simulink model "Guidance_PC_07Mar2013"  (Simulink 7.7)
settings: Solver=ode4  StartTime=0.0  StopTime=inf  FixedStep=sample_time  RelTol=1e-3
InitFcn:
  | sample_time=0.02;
undefined symbols (not defined in the file or in its folder): DiscIntNeverNeededParam
libraries: simulink x6, utility x1
(part 1 of 2)
settings Model: Creator=ttcl3  LastModifiedBy=Zhao Weihua
settings SolverCC: MaxConsecutiveMinStep=auto
settings DebuggingCC: MultiTaskRateTransMsg=warning

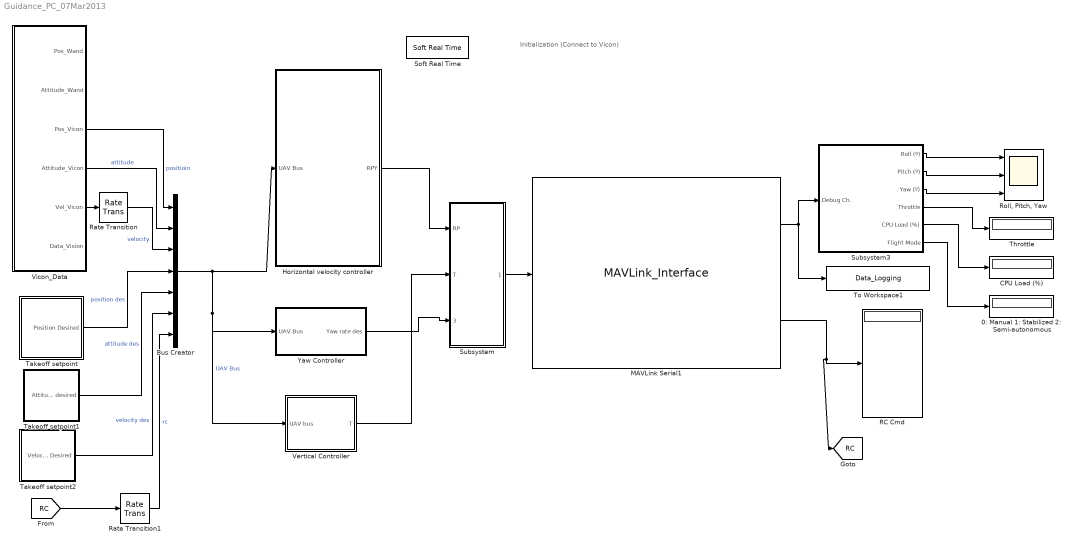
== system Guidance_PC_07Mar2013 ==
  note: Initialization
      | (Connect to Vicon)
  0: Manual 1: Stabilized 2: Semi-autonomous : Display
  Bus Creator : BusCreator  Inputs=7
  CPU Load (%) : Display
  Horizontal velocity controller : Subsystem
  MAVLink Serial1 : S-Function  FunctionName=MAVLink_Interface  Parameters=COM_Port,Baud_Rate,MSG_INPUT,MSG_OUTPUT  EnableBusSupport=off  mask{COM_Port='COM8', Baud_Rate=57600, HEART_BEAT=off, ATTITUDE_OUT=on, RAW_IMU=off, POSITION_OUT=off, VFR_HUD=off, RC_SCALED=on, SERVO_OUT_RAW=off, VICON_XYZ_RPY_Output=off, SET_MODE=off, DATA_STREAM=off, ATTITUDE_COMMAND=off, ATTITUDE_IN=off, GPS_RAW_IN=off, VFR_HUD_IN=off, VICON_XYZ_RPY=on, VICON_VEL=off, POSITION_DESIRED=off}
      mask prompts: COM_Port "COM Port"; Baud_Rate "Baud Rate"; HEART_BEAT "HEART BEAT"; ATTITUDE_OUT "ATTITUDE"; RAW_IMU "RAW IMU"; POSITION_OUT "GLOBAL POSITION"; VFR_HUD "VFR HUD"; RC_SCALED "RC CHANNELS SCALED"; SERVO_OUT_RAW "SERVO OUTPUT RAW"; VICON_XYZ_RPY_Output "VICON Output"; SET_MODE "SET MODE"; DATA_STREAM "REQUEST DATA STREAM"; ATTITUDE_COMMAND "ATTITUDE COMMAND"; ATTITUDE_IN "ATTITUDE (HIL)"; GPS_RAW_IN "GPS RAW (HIL)"; VFR_HUD_IN "AIRSPEED (HIL)"; VICON_XYZ_RPY "VICON POSITION"; VICON_VEL "VICON SPEED"; POSITION_DESIRED "Position Desired"
      mask init:
      | MSG_ID_NUM_INPUT = [uint8(11) uint8(66) uint8(59) uint8(30) uint8(32) uint8(73) uint8(104) uint8(103) uint8(50)];
      | MSG_ID_NAME_INPUT = [SET_MODE DATA_STREAM ATTITUDE_COMMAND ATTITUDE_IN GPS_RAW_IN VFR_HUD_IN VICON_XYZ_RPY VICON_VEL POSITION_DESIRED];
      | 
      | MSG_ID_NUM_OUTPUT = [uint8(0) uint8(30) uint8(27) uint8(73) uint8(74) uint8(34) uint8(37) uint8(104)];
      | MSG_ID_NAME_OUTPUT = [HEART_BEAT ATTITUDE_OUT RAW_IMU VFR_HUD POSITION_OUT RC_SCALED SERVO_OUT_RAW VICON_XYZ_RPY_Output];
      | 
      | idx_input = find(MSG_ID_NAME_INPUT);
      | MSG_INPUT = MSG_ID_NUM_INPUT(idx_input);
      | 
      | idx_output = find(MSG_ID_NAME_OUTPUT);
      | MSG_OUTPUT = MSG_ID_NUM_OUTPUT(idx_output);
      mask TabNameString: Setting,Setting,Output Message,Output Message,Output Message,Output Message,Output Message,Output Message,Output Message,Output Message,Input Message,Input Message,Input Message,Input Message,Input Message,Input Message,Input Message,Input Message,Input Message
      mask Display:
      | % Block image
      | image(imread('10-inch Quad Heat Map.png'));
      | 
      | %Label block
      | fprintf('MAVLink Serial\n%s\n%dbps', COM_Port,  Baud_Rate)
      | 
      | 
      | %Label input ports
      | 
      | in = 1;
      | if (SET_MODE == 1)
      |     port_label('input', in, 'SET MODE');
      |     in = in + 1;
      | end
      | if (DATA_STREAM == 1)
      |     port_label('input', in, 'REQUEST DATA STREAM');
      |     in = in + 1;
      | end
      | if (ATTITUDE_COMMAND == 1)
      |     port_label('input', in, 'ATTITUDE COMMAND');
      |     in = in + 1;
      | end
      | if (ATTITUDE_IN == 1)
      |     port_label('input', in, 'ATTITUDE (HIL)');
      |     in = in + 1;
      | end
      | if (GPS_RAW_IN == 1)
      |     port_label('input', in, 'GPS RAW (HIL)');
      |     in = in + 1;
      | end
      | if (VFR_HUD_IN == 1)
      |     port_label('input', in, 'AIRSPEED (HIL)');
      |     in = in + 1;
      | end
      | if (VICON_XYZ_RPY == 1)
      |     port_label('input', in, 'RPYT CMD');
      |     in = in + 1;
      | end
      | if (VICON_VEL == 1)
      |     port_label('input', in, 'VICON_VEL');
      |     in = in + 1;
      | end
      | 
      | if (POSITION_DESIRED == 1)
      |     port_label('input', in, 'POSITION_DESIRED');
      |     in = in + 1;
      | end
      | 
      | %Label output ports
      | 
      | out = 1;
      | if (HEART_BEAT == 1)
      |     port_label('output', out, 'HEART BEAT');
      |     out = out + 1;
      | end
      | if (ATTITUDE_OUT == 1)
      |     port_label('output', out, 'DEBUG');
      |     out = out + 1;
      | end
      | if (RAW_IMU == 1)
      |     port_label('output', out, 'RAW IMU');
      |     out = out + 1;
      | end
      | if (POSITION_OUT == 1)
      |     port_label('output', out, 'GLOBAL POSITION');
      |     out = out + 1;
      | end
      | if (VFR_HUD == 1)
      |     port_label('output', out, 'VFR HUD');
      |     out = out + 1;
      | end
      | if (RC_SCALED == 1)
      |     port_label('output', out, 'RC CMD');
      |     out = out + 1;
      | end
      | if (SERVO_OUT_RAW == 1)
      |     port_label('output', out, 'SERVO OUTPUT RAW');
      |     out = out + 1;
      | end
      | % weihua, vicon output
      | if (VICON_XYZ_RPY_Output == 1)
      |     port_label('output', out, 'VICON_XYZ_RPY');
      |     out = out + 1;
      | end
  RC Cmd : Display
  Rate Transition : RateTransition  OutPortSampleTime=sample_time
  Rate Transition1 : RateTransition  OutPortSampleTime=sample_time
  "Roll, Pitch, Yaw" : Scope  NumInputPorts=3
      settings: TickLabels=on  TimeRange=60  YMin=-1~-0.1~-1  YMax=1~0.1~1  SampleInput=on
  Soft Real Time : utility/Soft Real Time  x=0.6
  Subsystem : Subsystem
  Subsystem3 : Subsystem
  Takeoff setpoint : Subsystem
  Takeoff setpoint1 : Subsystem
  Takeoff setpoint2 : Subsystem
  Throttle : Display
  To Workspace1 : ToWorkspace  VariableName=Data_Logging  SampleTime=-1  SaveFormat=Structure With Time
  Vertical Controller : Subsystem
  Vicon_Data : Subsystem
  Yaw Controller : Subsystem
  tag scope: RC=global
  wires:
  MAVLink Serial1/2 -> RC Cmd/1, [RC]
  Subsystem3/1(Roll (º)) -> "Roll, Pitch, Yaw"/1
  Subsystem3/2(Pitch (º)) -> "Roll, Pitch, Yaw"/2
  Subsystem3/3(Yaw (º)) -> "Roll, Pitch, Yaw"/3
  Subsystem3/4(Throttle) -> Throttle/1
  Subsystem3/5(CPU Load (%)) -> CPU Load (%)/1
  Subsystem3/6(Flight Mode) -> 0: Manual 1: Stabilized 2: Semi-autonomous/1
  MAVLink Serial1/1 -> Subsystem3/1(Debug Ch.), To Workspace1/1
  Vicon_Data/5(Vel_Vicon) -> Rate Transition/1
  [RC] -> Rate Transition1/1
  Horizontal velocity controller/1(RPY) -> Subsystem/1(RP)
  Subsystem/1(XYZ RPY) -> MAVLink Serial1/1
  Vicon_Data/3(Pos_Vicon) -> Bus Creator/1  "positioin"
  Vicon_Data/4(Attitude_Vicon) -> Bus Creator/2  "attitude"
  Rate Transition/1 -> Bus Creator/3  "velocity"
  Takeoff setpoint/1(Position Desired) -> Bus Creator/4  "position des"
  Takeoff setpoint1/1(Attitude desired) -> Bus Creator/5  "attitude des"
  Takeoff setpoint2/1(Velocity Desired) -> Bus Creator/6  "velocity des"
  Rate Transition1/1 -> Bus Creator/7  "rc"
  Bus Creator/1 -> Horizontal velocity controller/1(UAV Bus), Yaw Controller/1(UAV Bus), Vertical Controller/1(UAV bus)  "UAV Bus"
  Yaw Controller/1(Yaw rate des) -> Subsystem/3(Yaw rate)
  Vertical Controller/1(T) -> Subsystem/2(T)

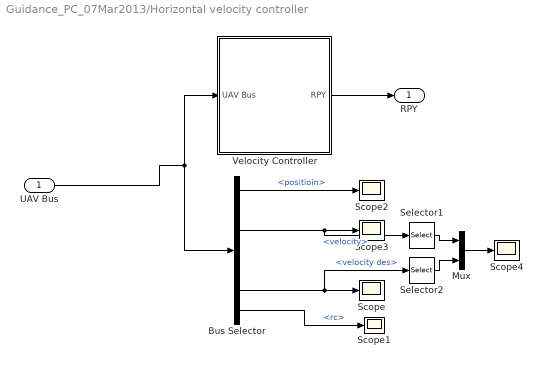
== system Guidance_PC_07Mar2013/Horizontal velocity controller ==
  UAV Bus : Inport
  Bus Selector : BusSelector  OutputSignals=positioin,attitude,velocity,position des,attitude des,velocity des,rc
  Mux : Mux  Inputs=2
  Scope{,1..4} (5 alike) : Scope
      Scope1 settings: SaveName=ScopeData2
      Scope2 settings: SaveName=ScopeData3
      Scope3 settings: SaveName=ScopeData6
      Scope4 settings: SaveName=ScopeData7
  Selector1 : Selector  InputPortWidth=3  IndexOptions=Index vector (dialog)  Indices=[2]  OutputSizes=1
  Selector2 : Selector  InputPortWidth=3  IndexOptions=Index vector (dialog)  Indices=[2]  OutputSizes=1
  Velocity Controller : Subsystem
  RPY : Outport
  wires:
  UAV Bus/1 -> Velocity Controller/1(UAV Bus), Bus Selector/1
  Velocity Controller/1(RPY) -> RPY/1
  Bus Selector/6 -> Scope/1, Selector2/1  "<velocity des>"
  Bus Selector/7 -> Scope1/1  "<rc>"
  Bus Selector/1 -> Scope2/1  "<positioin>"
  Bus Selector/3 -> Scope3/1, Selector1/1  "<velocity>"
  Selector1/1 -> Mux/1
  Selector2/1 -> Mux/2
  Mux/1 -> Scope4/1

== system Guidance_PC_07Mar2013/Subsystem ==
  note: 7x1 vector (usec, XYZRPY)
  RP : Inport
  T : Inport  Port=2
  Yaw rate : Inport  Port=3
  Mux1 : Mux  Inputs=3
  Mux2 : Mux  Inputs=3
  Mux3 : Mux  Inputs=2
  usec : Constant  Value=0
  XYZ RPY : Outport
  wires:
  Mux1/1 -> XYZ RPY/1
  usec/1 -> Mux1/1, Mux2/1, Mux2/2
  Mux2/1 -> Mux1/2
  T/1 -> Mux2/3
  RP/1 -> Mux3/1
  Yaw rate/1 -> Mux3/2
  Mux3/1 -> Mux1/3

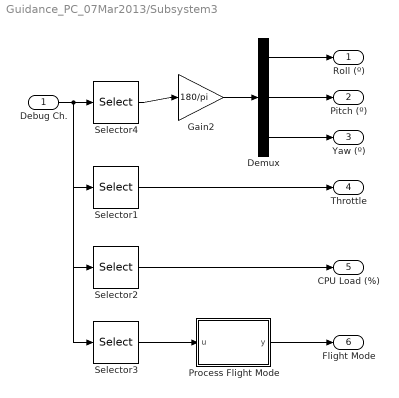
== system Guidance_PC_07Mar2013/Subsystem3 ==
  Debug Ch. : Inport
  Demux : Demux  Outputs=3
  Gain2 : Gain  Gain=180/pi
  Process Flight Mode : Stateflow chart  TreatAsAtomicUnit=on
  Selector1 : Selector  InputPortWidth=6  IndexOptions=Index vector (dialog)  Indices=4  OutputSizes=1
  Selector2 : Selector  InputPortWidth=6  IndexOptions=Index vector (dialog)  Indices=5  OutputSizes=1
  Selector3 : Selector  InputPortWidth=6  IndexOptions=Index vector (dialog)  Indices=6  OutputSizes=1
  Selector4 : Selector  InputPortWidth=6  IndexOptions=Index vector (dialog)  Indices=[1 2 3]  OutputSizes=1
  Roll (º) : Outport
  Pitch (º) : Outport  Port=2
  Yaw (º) : Outport  Port=3
  Throttle : Outport  Port=4
  CPU Load (%) : Outport  Port=5
  Flight Mode : Outport  Port=6
  wires:
  Selector4/1 -> Gain2/1
  Gain2/1 -> Demux/1
  Demux/1 -> Roll (º)/1
  Demux/2 -> Pitch (º)/1
  Debug Ch./1 -> Selector4/1, Selector1/1, Selector2/1, Selector3/1
  Demux/3 -> Yaw (º)/1
  Selector1/1 -> Throttle/1
  Selector2/1 -> CPU Load (%)/1
  Selector3/1 -> Process Flight Mode/1(u)
  Process Flight Mode/1(y) -> Flight Mode/1

== system Guidance_PC_07Mar2013/Takeoff setpoint ==
  Des_X : Constant  Value=0  SampleTime=sample_time
  Des_Y : Constant  Value=0  SampleTime=sample_time
  Des_Z : Constant  Value=-0.8  SampleTime=sample_time
  Mux3 : Mux  Inputs=3
  Position Desired : Outport
  wires:
  Des_X/1 -> Mux3/1
  Des_Y/1 -> Mux3/2
  Des_Z/1 -> Mux3/3
  Mux3/1 -> Position Desired/1

== system Guidance_PC_07Mar2013/Takeoff setpoint1 ==
  Mux3 : Mux  Inputs=3
  Pitch : Constant  Value=0  SampleTime=sample_time
  Roll : Constant  Value=0  SampleTime=sample_time
  Yaw : Constant  Value=0  OutDataTypeStr=double  SampleTime=sample_time
  Attitude desired : Outport
  wires:
  Mux3/1 -> Attitude desired/1
  Yaw/1 -> Mux3/3
  Pitch/1 -> Mux3/2
  Roll/1 -> Mux3/1

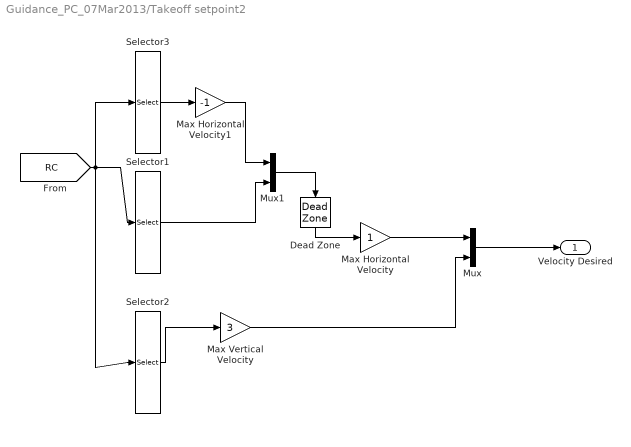
== system Guidance_PC_07Mar2013/Takeoff setpoint2 ==
  Dead Zone : DeadZone  LowerValue=-0.1  UpperValue=0.1  SaturateOnIntegerOverflow=on
  Max Horizontal Velocity : Gain  SampleTime=sample_time
  Max Horizontal Velocity1 : Gain  Gain=-1  OutDataTypeStr=double  SampleTime=sample_time
  Max Vertical Velocity : Gain  Gain=3  SampleTime=sample_time
  Mux : Mux  Inputs=2
  Mux1 : Mux  Inputs=2
  Selector1 : Selector  InputPortWidth=8  IndexOptions=Index vector (dialog)  Indices=[2]  OutputSizes=1
  Selector2 : Selector  InputPortWidth=8  IndexOptions=Index vector (dialog)  Indices=[1]  OutputSizes=1
  Selector3 : Selector  InputPortWidth=8  IndexOptions=Index vector (dialog)  Indices=[3]  OutputSizes=1
  Velocity Desired : Outport
  wires:
  [RC] -> Selector2/1, Selector1/1, Selector3/1
  Selector2/1 -> Max Vertical Velocity/1
  Mux/1 -> Velocity Desired/1
  Selector3/1 -> Max Horizontal Velocity1/1
  Selector1/1 -> Mux1/2
  Max Horizontal Velocity1/1 -> Mux1/1
  Mux1/1 -> Dead Zone/1
  Max Horizontal Velocity/1 -> Mux/1
  Max Vertical Velocity/1 -> Mux/2
  Dead Zone/1 -> Max Horizontal Velocity/1

== system Guidance_PC_07Mar2013/Vertical Controller ==
  UAV bus : Inport
  Bus Selector : BusSelector  OutputSignals=rc
  Selector2 : Selector  InputPortWidth=8  IndexOptions=Index vector (dialog)  Indices=[1]  OutputSizes=1
  T : Outport
  wires:
  UAV bus/1 -> Bus Selector/1
  Bus Selector/1 -> Selector2/1  "<rc>"
  Selector2/1 -> T/1

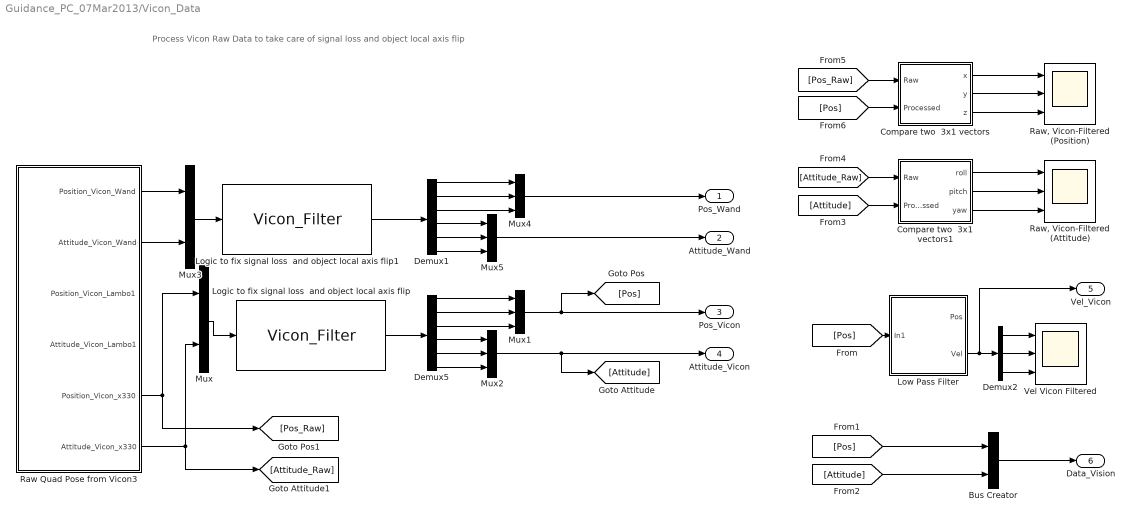
== system Guidance_PC_07Mar2013/Vicon_Data ==
  note: Process Vicon Raw Data to take care of signal loss and object local axis flip
  Bus Creator : BusCreator  Inputs=2
  Compare two  3x1 vectors : Subsystem
  Compare two  3x1 vectors1 : Subsystem
  Demux1 : Demux  Outputs=6
  Demux2 : Demux  Outputs=3
  Demux5 : Demux  Outputs=6
  Logic to fix signal loss  and object local axis flip : M-S-Function  FunctionName=Vicon_Filter
  Logic to fix signal loss  and object local axis flip1 : M-S-Function  FunctionName=Vicon_Filter
  Low Pass Filter : Subsystem
  Mux : Mux  Inputs=2
  Mux{1..2,4..5} (4 alike) : Mux  Inputs=3
  Mux3 : Mux  Inputs=2
  Raw Quad Pose from Vicon3 : Subsystem
  "Raw, Vicon-Filtered (Attitude)" : Scope  NumInputPorts=3
      settings: TimeRange=50  YMin=-3.14159~-1~-3.5  YMax=3.14159~1~3.5  SaveName=ScopeData4
  "Raw, Vicon-Filtered (Position)" : Scope  NumInputPorts=3
      settings: TimeRange=50  YMin=-2.09~2.281~-0.0655  YMax=-2.055~2.293~-0.063  SaveName=ScopeData10
  "Vel Vicon Filtered " : Scope  NumInputPorts=3
      settings: YMin=-0.7~-1~-9  YMax=0.4~7.5~0.5  SaveName=ScopeData5
  Pos_Wand : Outport
  Attitude_Wand : Outport  Port=2
  Pos_Vicon : Outport  Port=3
  Attitude_Vicon : Outport  Port=4
  Vel_Vicon : Outport  Port=5
  Data_Vision : Outport  Port=6
  wires:
  Demux2/1 -> "Vel Vicon Filtered "/1
  Demux2/2 -> "Vel Vicon Filtered "/2
  Demux2/3 -> "Vel Vicon Filtered "/3
  Compare two  3x1 vectors/1(x) -> "Raw, Vicon-Filtered (Position)"/1
  Compare two  3x1 vectors/2(y) -> "Raw, Vicon-Filtered (Position)"/2
  Low Pass Filter/2(Vel) -> Demux2/1, Vel_Vicon/1
  Mux/1 -> Logic to fix signal loss  and object local axis flip/1
  Logic to fix signal loss  and object local axis flip/1 -> Demux5/1
  Demux5/1 -> Mux1/1
  Demux5/2 -> Mux1/2
  Demux5/3 -> Mux1/3
  Demux5/4 -> Mux2/1
  Demux5/5 -> Mux2/2
  Demux5/6 -> Mux2/3
  Mux2/1 -> Attitude_Vicon/1, [Attitude]
  [Pos] -> Low Pass Filter/1(In1)
  Compare two  3x1 vectors/3(z) -> "Raw, Vicon-Filtered (Position)"/3
  Compare two  3x1 vectors1/1(roll) -> "Raw, Vicon-Filtered (Attitude)"/1
  Compare two  3x1 vectors1/2(pitch) -> "Raw, Vicon-Filtered (Attitude)"/2
  Mux1/1 -> Pos_Vicon/1, [Pos]
  Compare two  3x1 vectors1/3(yaw) -> "Raw, Vicon-Filtered (Attitude)"/3
  [Attitude_Raw] -> Compare two  3x1 vectors1/1(Raw)
  [Attitude] -> Compare two  3x1 vectors1/2(Processed)
  [Pos_Raw] -> Compare two  3x1 vectors/1(Raw)
  [Pos] -> Compare two  3x1 vectors/2(Processed)
  [Pos] -> Bus Creator/1
  [Attitude] -> Bus Creator/2
  Bus Creator/1 -> Data_Vision/1
  Mux3/1 -> Logic to fix signal loss  and object local axis flip1/1
  Logic to fix signal loss  and object local axis flip1/1 -> Demux1/1
  Demux1/1 -> Mux4/1
  Demux1/2 -> Mux4/2
  Demux1/3 -> Mux4/3
  Demux1/4 -> Mux5/1
  Demux1/5 -> Mux5/2
  Demux1/6 -> Mux5/3
  Mux5/1 -> Attitude_Wand/1
  Mux4/1 -> Pos_Wand/1
  Raw Quad Pose from Vicon3/1(Position_Vicon_Wand) -> Mux3/1
  Raw Quad Pose from Vicon3/2(Attitude_Vicon_Wand) -> Mux3/2
  Raw Quad Pose from Vicon3/5(Position_Vicon_x330) -> Mux/1, [Pos_Raw]
  Raw Quad Pose from Vicon3/6(Attitude_Vicon_x330) -> Mux/2, [Attitude_Raw]

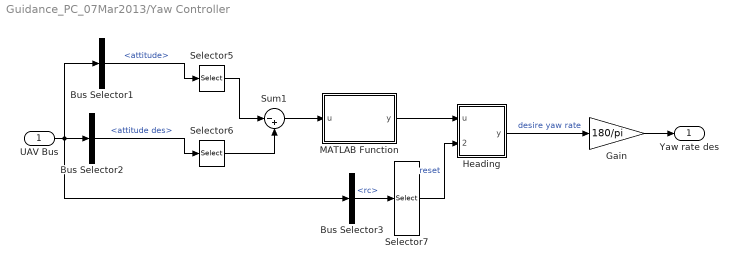
== system Guidance_PC_07Mar2013/Yaw Controller ==
  UAV Bus : Inport
  Bus Selector1 : BusSelector  OutputSignals=attitude
  Bus Selector2 : BusSelector  OutputSignals=attitude des
  Bus Selector3 : BusSelector  OutputSignals=rc
  Gain : Gain  Gain=180/pi
  Heading : Subsystem  AncestorBlock=simulink/Continuous/PID Controller  DialogController=pidpack.PIDConfig.pidDDGCreate  DialogControllerArgs=DataTag1  mask(PID 1dof){Controller=PI, TimeDomain=Discrete-time, SampleTime=sample_time, IntegratorMethod=Trapezoidal, FilterMethod=Trapezoidal, Form=Parallel, P=2, I=1, D=0, N=100, InitialConditionSource=internal, InitialConditionForIntegrator=0, InitialConditionForFilter=0, ExternalReset=rising, IgnoreLimit=off, ZeroCross=on, LimitOutput=on, UpperSaturationLimit=300*pi/180, LowerSaturationLimit=-300*pi/180, LinearizeAsGain=off, AntiWindupMode=none, Kb=1, TrackingMode=off, Kt=1, RndMeth=Floor, SaturateOnIntegerOverflow=off, LockScale=off, PParamMin=[], PParamMax=[], PParamDataTypeStr=Inherit: Inherit via internal rule, IParamMin=[], IParamMax=[], IParamDataTypeStr=Inherit: Inherit via internal rule, DParamMin=[], DParamMax=[], DParamDataTypeStr=Inherit: Inherit via internal rule, NParamMin=[], NParamMax=[], NParamDataTypeStr=Inherit: Inherit via internal rule, KbParamMin=[], KbParamMax=[], KbParamDataTypeStr=Inherit: Inherit via internal rule, KtParamMin=[], KtParamMax=[], KtParamDataTypeStr=Inherit: Inherit via internal rule, POutMin=[], POutMax=[], POutDataTypeStr=Inherit: Inherit via internal rule, IOutMin=[], IOutMax=[], IOutDataTypeStr=Inherit: Inherit via internal rule, DOutMin=[], DOutMax=[], DOutDataTypeStr=Inherit: Inherit via internal rule, NOutMin=[], NOutMax=[], NOutDataTypeStr=Inherit: Inherit via internal rule, KbOutMin=[], KbOutMax=[], KbOutDataTypeStr=Inherit: Inherit via internal rule, KtOutMin=[], KtOutMax=[], KtOutDataTypeStr=Inherit: Inherit via internal rule, IntegratorOutMin=[], IntegratorOutMax=[], IntegratorOutDataTypeStr=Inherit: Inherit via internal rule, FilterOutMin=[], FilterOutMax=[], FilterOutDataTypeStr=Inherit: Inherit via internal rule, SumOutMin=[], SumOutMax=[], SumOutDataTypeStr=Inherit: Inherit via internal rule, SumI1OutMin=[], SumI1OutMax=[], SumI1OutDataTypeStr=Inherit: Inherit via internal rule, SumI2OutMin=[], SumI2OutMax=[], SumI2OutDataTypeStr=Inherit: Inherit via internal rule, SumI3OutMin=[], SumI3OutMax=[], SumI3OutDataTypeStr=Inherit: Inherit via internal rule, SumDOutMin=[], SumDOutMax=[], SumDOutDataTypeStr=Inherit: Inherit via internal rule, SumAccumDataTypeStr=Inherit: Inherit via internal rule, SumI1AccumDataTypeStr=Inherit: Inherit via internal rule, SumI2AccumDataTypeStr=Inherit: Inherit via internal rule, SumI3AccumDataTypeStr=Inherit: Inherit via internal rule, SumDAccumDataTypeStr=Inherit: Inherit via internal rule, SaturationOutMin=[], SaturationOutMax=[], SaturationOutDataTypeStr=Inherit: Same as input, IntegratorContinuousStateAttributes='', IntegratorStateIdentifier=, IntegratorStateMustResolveToSignalObject=off, IntegratorRTWStateStorageClass=Auto, IntegratorRTWStateStorageTypeQualifier=, FilterContinuousStateAttributes='', FilterStateIdentifier=, FilterStateMustResolveToSignalObject=off, FilterRTWStateStorageClass=Auto, FilterRTWStateStorageTypeQualifier=}
      mask prompts: TimeDomain "Time domain:"; SampleTime "Sample time (-1 for inherited):"; IntegratorMethod "Integrator method:"; FilterMethod "Filter method:"; P "Proportional (P):"; I "Integral (I):"; D "Derivative (D):"; N "Filter coefficient (N):"; InitialConditionSource "Source:"; InitialConditionForIntegrator "Integrator:"; InitialConditionForFilter "Filter:"; ExternalReset "External reset:"; IgnoreLimit "Ignore reset when linearizing"; ZeroCross "Enable zero-crossing detection"; LimitOutput "Limit output"; UpperSaturationLimit "Upper saturation limit:"; LowerSaturationLimit "Lower saturation limit:"; LinearizeAsGain "Ignore saturation when linearizing"; AntiWindupMode "Anti-windup method:"; Kb "Back-calculation coefficient (Kb):"; TrackingMode "Enable tracking mode"; Kt "Tracking coefficient (Kt):"; RndMeth "Integer rounding mode:"; SaturateOnIntegerOverflow "Saturate on integer overflow"; LockScale "Lock data type settings against changes by the fixed-point tools"; PParamMin "P parameter minimum:"; PParamMax "P parameter maximum:"; PParamDataTypeStr "P parameter:"; IParamMin "I parameter minimum:"; IParamMax "I parameter maximum:"; IParamDataTypeStr "I parameter:"; DParamMin "D parameter minimum:"; DParamMax "D parameter maximum:"; DParamDataTypeStr "D parameter:"; NParamMin "N parameter minimum:"; NParamMax "N parameter maximum:"; NParamDataTypeStr "N parameter:"; KbParamMin "Kb parameter minimum:"; KbParamMax "Kb parameter maximum:"; KbParamDataTypeStr "Kb parameter:"; KtParamMin "Kt parameter minimum:"; KtParamMax "Kt parameter maximum:"; KtParamDataTypeStr "Kt parameter:"; POutMin "P product output minimum:"; POutMax "P product output maximum:"; POutDataTypeStr "P product output:"; IOutMin "I product output minimum:"; IOutMax "I product output maximum:"; IOutDataTypeStr "I product output:"; DOutMin "D product output minimum:"; DOutMax "D product output maximum:"; DOutDataTypeStr "D product output:"; NOutMin "N product output minimum:"; NOutMax "N product output maximum:"; NOutDataTypeStr "N product output:"; KbOutMin "Kb product output minimum:"; KbOutMax "Kb product output maximum:"; KbOutDataTypeStr "Kb product output:"; KtOutMin "Kt product output minimum:"; KtOutMax "Kt product output maximum:"; KtOutDataTypeStr "Kt product output:"; IntegratorOutMin "Integrator output minimum:"; IntegratorOutMax "Integrator output maximum:"; IntegratorOutDataTypeStr "Integrator output:"; FilterOutMin "Filter output minimum:"; FilterOutMax "Filter output maximum:"; FilterOutDataTypeStr "Filter output:"; SumOutMin "Sum output minimum:"; SumOutMax "Sum output maximum:"; SumOutDataTypeStr "Sum output:"; SumI1OutMin "SumI1 output minimum:"; SumI1OutMax "SumI1 output maximum:"; SumI1OutDataTypeStr "SumI1 output:"; SumI2OutMin "SumI2 output minimum:"; SumI2OutMax "SumI2 output maximum:"; SumI2OutDataTypeStr "SumI2 output:"; SumI3OutMin "SumI3 output minimum:"; SumI3OutMax "SumI3 output maximum:"; SumI3OutDataTypeStr "SumI3 output:"; SumDOutMin "SumD output minimum:"; SumDOutMax "SumD output maximum:"; SumDOutDataTypeStr "SumD output:"; SumAccumDataTypeStr "Accumulator of Sum:"; SumI1AccumDataTypeStr "Accumulator of SumI1:"; SumI2AccumDataTypeStr "Accumulator of SumI2:"; SumI3AccumDataTypeStr "Accumulator of SumI3:"; SumDAccumDataTypeStr "Accumulator of SumD:"; SaturationOutMin "Saturation output minimum:"; SaturationOutMax "Saturation output maximum:"; SaturationOutDataTypeStr "Saturation output:"; IntegratorContinuousStateAttributes "State name: (e.g., 'position')"; IntegratorStateIdentifier "State name:"; IntegratorStateMustResolveToSignalObject "State name must resolve to Simulink signal object"; IntegratorRTWStateStorageClass "Code generation storage class:"; IntegratorRTWStateStorageTypeQualifier "Code generation storage type qualifier:"; FilterContinuousStateAttributes "State name: (e.g., 'position')"; FilterStateIdentifier "State name:"; FilterStateMustResolveToSignalObject "State name must resolve to Simulink signal object"; FilterRTWStateStorageClass "Code generation storage class:"; FilterRTWStateStorageTypeQualifier "Code generation storage type qualifier:"
      mask help: This block implements continuous- and discrete-time PID control algorithms and includes advanced features such as anti-windup, external reset, and signal tracking. You can tune the PID gains automatically using the 'Tune...' button (requires Simulink Control Design).
      mask init:
      | pidpack.PIDConfig.configPID(gcbh);
      settings: DeleteFcn=pidpack.PIDConfig.closeTuner(gcbh)  ModelCloseFcn=pidpack.PIDConfig.closeTuner(gcbh)  NameChangeFcn=pidpack.PIDConfig.updateTunerName(gcbh)
      mask StyleString: popup(PID|PI|PD|P|I),popup(Continuous-time|Discrete-time),edit,popup(Forward Euler|Backward Euler|Trapezoidal),popup(Forward Euler|Backward Euler|Trapezoidal),popup(Ideal|Parallel),edit,edit,edit,edit,popup(internal|external),edit,edit,popup(none|rising|falling|either|level),checkbox,checkbox,checkbox,edit,edit,checkbox,popup(none|back-calculation|clamping),edit,checkbox,edit,popup(Ceiling|Convergent|Floor|Nearest|Round|Simplest|Zero),checkbox,checkbox,min,max,unidt({a=30|28|29|}{i=Inherit: Inherit via internal rule|Inherit: Same as input}{b=double|single|int8|uint8|int16|uint16|int32|uint32}{s=UDTBinaryPointMode|UDTSlopeBiasMode|UDTBestPrecisionMode}{g=UDTSignedSign|UDTUnsignedSign}),min,max,unidt({a=33|31|32|}{i=Inherit: Inherit via internal rule|Inherit: Same as input}{b=double|single|int8|uint8|int16|uint16|int32|uint32}{s=UDTBinaryPointMode|UDTSlopeBiasMode|UDTBestPrecisionMode}{g=UDTSignedSign|UDTUnsignedSign}),min,max,unidt({a=36|34|35|}{i=Inherit: Inherit via internal rule|Inherit: Same as input}{b=double|single|int8|uint8|int16|uint16|int32|uint32}{s=UDTBinaryPointMode|UDTSlopeBiasMode|UDTBestPrecisionMode}{g=UDTSignedSign|UDTUnsignedSign}),min,max,unidt({a=39|37|38|}{i=Inherit: Inherit via internal rule|Inherit: Same as input}{b=double|single|int8|uint8|int16|uint16|int32|uint32}{s=UDTBinaryPointMode|UDTSlopeBiasMode|UDTBestPrecisionMode}{g=UDTSignedSign|UDTUnsignedSign}),min,max,unidt({a=42|40|41|}{i=Inherit: Inherit via internal rule|Inherit: Same as input}{b=double|single|int8|uint8|int16|uint16|int32|uint32}{s=UDTBinaryPointMode|UDTSlopeBiasMode|UDTBestPrecisionMode}{g=UDTSignedSign|UDTUnsignedSign}),min,max,unidt({a=45|43|44|}{i=Inherit: Inherit via internal rule|Inherit: Same as input}{b=double|single|int8|uint8|int16|uint16|int32|uint32}{s=UDTBinaryPointMode|UDTSlopeBiasMode|UDTBestPrecisionMode}{g=UDTSignedSign|UDTUnsignedSign}),min,max,unidt({a=48|46|47|}{i=Inherit: Inherit via internal rule|Inherit: Inherit via back propagation|Inherit: Same as input}{b=double|single|int8|uint8|int16|uint16|int32|uint32}{s=UDTBinaryPointMode|UDTSlopeBiasMode}{g=UDTSignedSign|UDTUnsignedSign}),min,max,unidt({a=51|49|50|}{i=Inherit: Inherit via internal rule|Inherit: Inherit via back propagation|Inherit: Same as input}{b=double|single|int8|uint8|int16|uint16|int32|uint32}{s=UDTBinaryPointMode|UDTSlopeBiasMode}{g=UDTSignedSign|UDTUnsignedSign}),min,max,unidt({a=54|52|53|}{i=Inherit: Inherit via internal rule|Inherit: Inherit via back propagation|Inherit: Same as input}{b=double|single|int8|uint8|int16|uint16|int32|uint32}{s=UDTBinaryPointMode|UDTSlopeBiasMode}{g=UDTSignedSign|UDTUnsignedSign}),min,max,unidt({a=57|55|56|}{i=Inherit: Inherit via internal rule|Inherit: Inherit via back propagation|Inherit: Same as input}{b=double|single|int8|uint8|int16|uint16|int32|uint32}{s=UDTBinaryPointMode|UDTSlopeBiasMode}{g=UDTSignedSign|UDTUnsignedSign}),min,max,unidt({a=60|58|59|}{i=Inherit: Inherit via internal rule|Inherit: Inherit via back propagation|Inherit: Same as input}{b=double|single|int8|uint8|int16|uint16|int32|uint32}{s=UDTBinaryPointMode|UDTSlopeBiasMode}{g=UDTSignedSign|UDTUnsignedSign}),min,max,unidt({a=63|61|62|}{i=Inherit: Inherit via internal rule|Inherit: Inherit via back propagation|Inherit: Same as input}{b=double|single|int8|uint8|int16|uint16|int32|uint32}{s=UDTBinaryPointMode|UDTSlopeBiasMode}{g=UDTSignedSign|UDTUnsignedSign}),min,max,unidt({a=66|64|65|}{i=Inherit: Inherit via internal rule|Inherit: Inherit via back propagation}{b=double|single|int8|uint8|int16|uint16|int32|uint32}{s=UDTBinaryPointMode|UDTSlopeBiasMode}{g=UDTSignedSign|UDTUnsignedSign}),min,max,unidt({a=69|67|68|}{i=Inherit: Inherit via internal rule|Inherit: Inherit via back propagation}{b=double|single|int8|uint8|int16|uint16|int32|uint32}{s=UDTBinaryPointMode|UDTSlopeBiasMode}{g=UDTSignedSign|UDTUnsignedSign}),min,max,unidt({a=72|70|71|}{i=Inherit: Inherit via internal rule|Inherit: Inherit via back propagation|Inherit: Same as first input|Inherit: Same as accumulator}{b=double|single|int8|uint8|int16|uint16|int32|uint32}{s=UDTBinaryPointMode|UDTSlopeBiasMode}{g=UDTSignedSign|UDTUnsignedSign}),min,max,unidt({a=75|73|74|}{i=Inherit: Inherit via internal rule|Inherit: Inherit via back propagation|Inherit: Same as first input|Inherit: Same as accumulator}{b=double|single|int8|uint8|int16|uint16|int32|uint32}{s=UDTBinaryPointMode|UDTSlopeBiasMode}{g=UDTSignedSign|UDTUnsignedSign}),min,max,unidt({a=78|76|77|}{i=Inherit: Inherit via internal rule|Inherit: Inherit via back propagation|Inherit: Same as first input|Inherit: Same as accumulator}{b=double|single|int8|uint8|int16|uint16|int32|uint32}{s=UDTBinaryPointMode|UDTSlopeBiasMode}{g=UDTSignedSign|UDTUnsignedSign}),min,max,unidt({a=81|79|80|}{i=Inherit: Inherit via internal rule|Inherit: Inherit via back propagation|Inherit: Same as first input|Inherit: Same as accumulator}{b=double|single|int8|uint8|int16|uint16|int32|uint32}{s=UDTBinaryPointMode|UDTSlopeBiasMode}{g=UDTSignedSign|UDTUnsignedSign}),min,max,unidt({a=84|82|83|}{i=Inherit: Inherit via internal rule|Inherit: Inherit via back propagation|Inherit: Same as first input|Inherit: Same as accumulator}{b=double|single|int8|uint8|int16|uint16|int32|uint32}{s=UDTBinaryPointMode|UDTSlopeBiasMode}{g=UDTSignedSign|UDTUnsignedSign}),unidt({a=85|||}{i=Inherit: Inherit via internal rule|Inherit: Same as first input}{b=double|single|int8|uint8|int16|uint16|int32|uint32}{s=UDTBinaryPointMode|UDTSlopeBiasMode}{g=UDTSignedSign|UDTUnsignedSign}),unidt({a=86|||}{i=Inherit: Inherit via internal rule|Inherit: Same as first input}{b=double|single|int8|uint8|int16|uint16|int32|uint32}{s=UDTBinaryPointMode|UDTSlopeBiasMode}{g=UDTSignedSign|UDTUnsignedSign}),unidt({a=87|||}{i=Inherit: Inherit via internal rule|Inherit: Same as first input}{b=double|single|int8|uint8|int16|uint16|int32|uint32}{s=UDTBinaryPointMode|UDTSlopeBiasMode}{g=UDTSignedSign|UDTUnsignedSign}),unidt({a=88|||}{i=Inherit: Inherit via internal rule|Inherit: Same as first input}{b=double|single|int8|uint8|int16|uint16|int32|uint32}{s=UDTBinaryPointMode|UDTSlopeBiasMode}{g=UDTSignedSign|UDTUnsignedSign}),unidt({a=89|||}{i=Inherit: Inherit via internal rule|Inherit: Same as first input}{b=double|single|int8|uint8|int16|uint16|int32|uint32}{s=UDTBinaryPointMode|UDTSlopeBiasMode}{g=UDTSignedSign|UDTUnsignedSign}),min,max,unidt({a=92|90|91|}{i=Inherit: Inherit via back propagation|Inherit: Same as input}{b=double|single|int8|uint8|int16|uint16|int32|uint32}{s=UDTBinaryPointMode|UDTSlopeBiasMode}{g=UDTSignedSign|UDTUnsignedSign}),edit,edit,checkbox,popup(Auto|ExportedGlobal|ImportedExtern|ImportedExternPointer),edit,edit,edit,checkbox,popup(Auto|ExportedGlobal|ImportedExtern|ImportedExternPointer),edit
      mask Display:
      | disp('PI(z)')
      | port_label('input',1, '');
      | port_label('output',1, '');plot([0 4 4 7]+2,[0 0 8 8]+8);
      | plot([1 4 6]+2,[3 6 3]+8);
      | plot([0 4 6 10]+32,[0 0 8 8]+18);
  MATLAB Function : Stateflow chart  TreatAsAtomicUnit=on
  Selector5 : Selector  InputPortWidth=3  IndexOptions=Index vector (dialog)  Indices=[3]  OutputSizes=1
  Selector6 : Selector  InputPortWidth=3  IndexOptions=Index vector (dialog)  Indices=[3]  OutputSizes=1
  Selector7 : Selector  InputPortWidth=8  IndexOptions=Index vector (dialog)  Indices=[5]  OutputSizes=1
  Sum1 : Sum  Inputs=|-+
  Yaw rate des : Outport
  wires:
  Bus Selector2/1 -> Selector6/1  "<attitude des>"
  Selector6/1 -> Sum1/2
  Sum1/1 -> MATLAB Function/1(u)
  MATLAB Function/1(y) -> Heading/1(u)
  UAV Bus/1 -> Bus Selector2/1, Bus Selector3/1, Bus Selector1/1
  Bus Selector1/1 -> Selector5/1  "<attitude>"
  Heading/1(y) -> Gain/1  "desire yaw rate"
  Selector7/1 -> Heading/2(RESET)  "reset"
  Bus Selector3/1 -> Selector7/1  "<rc>"
  Selector5/1 -> Sum1/1
  Gain/1 -> Yaw rate des/1

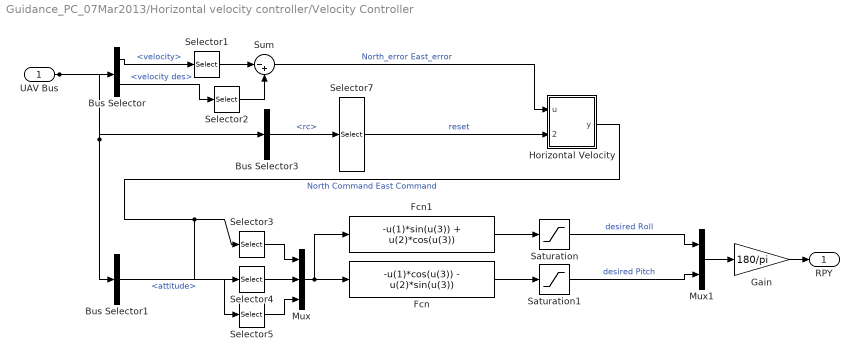
== system Guidance_PC_07Mar2013/Horizontal velocity controller/Velocity Controller ==
  UAV Bus : Inport
  Bus Selector : BusSelector  OutputSignals=velocity,velocity des
  Bus Selector1 : BusSelector  OutputSignals=attitude
  Bus Selector3 : BusSelector  OutputSignals=rc
  Fcn : Fcn  Expr=-u(1)*cos(u(3)) - u(2)*sin(u(3))
  Fcn1 : Fcn  Expr=-u(1)*sin(u(3)) + u(2)*cos(u(3))
  Gain : Gain  Gain=180/pi
  Horizontal Velocity : Subsystem  AncestorBlock=simulink/Continuous/PID Controller  DialogController=pidpack.PIDConfig.pidDDGCreate  DialogControllerArgs=DataTag0  mask(PID 1dof){Controller=PI, TimeDomain=Discrete-time, SampleTime=sample_time, IntegratorMethod=Trapezoidal, FilterMethod=Trapezoidal, Form=Parallel, P=0.14, I=0.03, D=0, N=100, InitialConditionSource=internal, InitialConditionForIntegrator=0, InitialConditionForFilter=0, ExternalReset=rising, IgnoreLimit=off, ZeroCross=on, LimitOutput=on, UpperSaturationLimit=30*pi/180, LowerSaturationLimit=-30*pi/180, LinearizeAsGain=off, AntiWindupMode=none, Kb=1, TrackingMode=off, Kt=1, RndMeth=Floor, SaturateOnIntegerOverflow=off, LockScale=off, PParamMin=[], PParamMax=[], PParamDataTypeStr=double, IParamMin=[], IParamMax=[], IParamDataTypeStr=double, DParamMin=[], DParamMax=[], DParamDataTypeStr=Inherit: Inherit via internal rule, NParamMin=[], NParamMax=[], NParamDataTypeStr=Inherit: Inherit via internal rule, KbParamMin=[], KbParamMax=[], KbParamDataTypeStr=Inherit: Inherit via internal rule, KtParamMin=[], KtParamMax=[], KtParamDataTypeStr=Inherit: Inherit via internal rule, POutMin=[], POutMax=[], POutDataTypeStr=double, IOutMin=[], IOutMax=[], IOutDataTypeStr=double, DOutMin=[], DOutMax=[], DOutDataTypeStr=Inherit: Inherit via internal rule, NOutMin=[], NOutMax=[], NOutDataTypeStr=Inherit: Inherit via internal rule, KbOutMin=[], KbOutMax=[], KbOutDataTypeStr=Inherit: Inherit via internal rule, KtOutMin=[], KtOutMax=[], KtOutDataTypeStr=Inherit: Inherit via internal rule, IntegratorOutMin=[], IntegratorOutMax=[], IntegratorOutDataTypeStr=double, FilterOutMin=[], FilterOutMax=[], FilterOutDataTypeStr=Inherit: Inherit via internal rule, SumOutMin=[], SumOutMax=[], SumOutDataTypeStr=double, SumI1OutMin=[], SumI1OutMax=[], SumI1OutDataTypeStr=Inherit: Inherit via internal rule, SumI2OutMin=[], SumI2OutMax=[], SumI2OutDataTypeStr=Inherit: Inherit via internal rule, SumI3OutMin=[], SumI3OutMax=[], SumI3OutDataTypeStr=Inherit: Inherit via internal rule, SumDOutMin=[], SumDOutMax=[], SumDOutDataTypeStr=Inherit: Inherit via internal rule, SumAccumDataTypeStr=double, SumI1AccumDataTypeStr=Inherit: Inherit via internal rule, SumI2AccumDataTypeStr=Inherit: Inherit via internal rule, SumI3AccumDataTypeStr=Inherit: Inherit via internal rule, SumDAccumDataTypeStr=Inherit: Inherit via internal rule, SaturationOutMin=[], SaturationOutMax=[], SaturationOutDataTypeStr=double, IntegratorContinuousStateAttributes='', IntegratorStateIdentifier=, IntegratorStateMustResolveToSignalObject=off, IntegratorRTWStateStorageClass=Auto, IntegratorRTWStateStorageTypeQualifier=, FilterContinuousStateAttributes='', FilterStateIdentifier=, FilterStateMustResolveToSignalObject=off, FilterRTWStateStorageClass=Auto, FilterRTWStateStorageTypeQualifier=}
      mask prompts: TimeDomain "Time domain:"; SampleTime "Sample time (-1 for inherited):"; IntegratorMethod "Integrator method:"; FilterMethod "Filter method:"; P "Proportional (P):"; I "Integral (I):"; D "Derivative (D):"; N "Filter coefficient (N):"; InitialConditionSource "Source:"; InitialConditionForIntegrator "Integrator:"; InitialConditionForFilter "Filter:"; ExternalReset "External reset:"; IgnoreLimit "Ignore reset when linearizing"; ZeroCross "Enable zero-crossing detection"; LimitOutput "Limit output"; UpperSaturationLimit "Upper saturation limit:"; LowerSaturationLimit "Lower saturation limit:"; LinearizeAsGain "Ignore saturation when linearizing"; AntiWindupMode "Anti-windup method:"; Kb "Back-calculation coefficient (Kb):"; TrackingMode "Enable tracking mode"; Kt "Tracking coefficient (Kt):"; RndMeth "Integer rounding mode:"; SaturateOnIntegerOverflow "Saturate on integer overflow"; LockScale "Lock data type settings against changes by the fixed-point tools"; PParamMin "P parameter minimum:"; PParamMax "P parameter maximum:"; PParamDataTypeStr "P parameter:"; IParamMin "I parameter minimum:"; IParamMax "I parameter maximum:"; IParamDataTypeStr "I parameter:"; DParamMin "D parameter minimum:"; DParamMax "D parameter maximum:"; DParamDataTypeStr "D parameter:"; NParamMin "N parameter minimum:"; NParamMax "N parameter maximum:"; NParamDataTypeStr "N parameter:"; KbParamMin "Kb parameter minimum:"; KbParamMax "Kb parameter maximum:"; KbParamDataTypeStr "Kb parameter:"; KtParamMin "Kt parameter minimum:"; KtParamMax "Kt parameter maximum:"; KtParamDataTypeStr "Kt parameter:"; POutMin "P product output minimum:"; POutMax "P product output maximum:"; POutDataTypeStr "P product output:"; IOutMin "I product output minimum:"; IOutMax "I product output maximum:"; IOutDataTypeStr "I product output:"; DOutMin "D product output minimum:"; DOutMax "D product output maximum:"; DOutDataTypeStr "D product output:"; NOutMin "N product output minimum:"; NOutMax "N product output maximum:"; NOutDataTypeStr "N product output:"; KbOutMin "Kb product output minimum:"; KbOutMax "Kb product output maximum:"; KbOutDataTypeStr "Kb product output:"; KtOutMin "Kt product output minimum:"; KtOutMax "Kt product output maximum:"; KtOutDataTypeStr "Kt product output:"; IntegratorOutMin "Integrator output minimum:"; IntegratorOutMax "Integrator output maximum:"; IntegratorOutDataTypeStr "Integrator output:"; FilterOutMin "Filter output minimum:"; FilterOutMax "Filter output maximum:"; FilterOutDataTypeStr "Filter output:"; SumOutMin "Sum output minimum:"; SumOutMax "Sum output maximum:"; SumOutDataTypeStr "Sum output:"; SumI1OutMin "SumI1 output minimum:"; SumI1OutMax "SumI1 output maximum:"; SumI1OutDataTypeStr "SumI1 output:"; SumI2OutMin "SumI2 output minimum:"; SumI2OutMax "SumI2 output maximum:"; SumI2OutDataTypeStr "SumI2 output:"; SumI3OutMin "SumI3 output minimum:"; SumI3OutMax "SumI3 output maximum:"; SumI3OutDataTypeStr "SumI3 output:"; SumDOutMin "SumD output minimum:"; SumDOutMax "SumD output maximum:"; SumDOutDataTypeStr "SumD output:"; SumAccumDataTypeStr "Accumulator of Sum:"; SumI1AccumDataTypeStr "Accumulator of SumI1:"; SumI2AccumDataTypeStr "Accumulator of SumI2:"; SumI3AccumDataTypeStr "Accumulator of SumI3:"; SumDAccumDataTypeStr "Accumulator of SumD:"; SaturationOutMin "Saturation output minimum:"; SaturationOutMax "Saturation output maximum:"; SaturationOutDataTypeStr "Saturation output:"; IntegratorContinuousStateAttributes "State name: (e.g., 'position')"; IntegratorStateIdentifier "State name:"; IntegratorStateMustResolveToSignalObject "State name must resolve to Simulink signal object"; IntegratorRTWStateStorageClass "Code generation storage class:"; IntegratorRTWStateStorageTypeQualifier "Code generation storage type qualifier:"; FilterContinuousStateAttributes "State name: (e.g., 'position')"; FilterStateIdentifier "State name:"; FilterStateMustResolveToSignalObject "State name must resolve to Simulink signal object"; FilterRTWStateStorageClass "Code generation storage class:"; FilterRTWStateStorageTypeQualifier "Code generation storage type qualifier:"
      mask help: This block implements continuous- and discrete-time PID control algorithms and includes advanced features such as anti-windup, external reset, and signal tracking. You can tune the PID gains automatically using the 'Tune...' button (requires Simulink Control Design).
      mask init:
      | pidpack.PIDConfig.configPID(gcbh);
      settings: DeleteFcn=pidpack.PIDConfig.closeTuner(gcbh)  ModelCloseFcn=pidpack.PIDConfig.closeTuner(gcbh)  NameChangeFcn=pidpack.PIDConfig.updateTunerName(gcbh)
      mask StyleString: popup(PID|PI|PD|P|I),popup(Continuous-time|Discrete-time),edit,popup(Forward Euler|Backward Euler|Trapezoidal),popup(Forward Euler|Backward Euler|Trapezoidal),popup(Ideal|Parallel),edit,edit,edit,edit,popup(internal|external),edit,edit,popup(none|rising|falling|either|level),checkbox,checkbox,checkbox,edit,edit,checkbox,popup(none|back-calculation|clamping),edit,checkbox,edit,popup(Ceiling|Convergent|Floor|Nearest|Round|Simplest|Zero),checkbox,checkbox,min,max,unidt({a=30|28|29|}{i=Inherit: Inherit via internal rule|Inherit: Same as input}{b=double|single|int8|uint8|int16|uint16|int32|uint32}{s=UDTBinaryPointMode|UDTSlopeBiasMode|UDTBestPrecisionMode}{g=UDTSignedSign|UDTUnsignedSign}),min,max,unidt({a=33|31|32|}{i=Inherit: Inherit via internal rule|Inherit: Same as input}{b=double|single|int8|uint8|int16|uint16|int32|uint32}{s=UDTBinaryPointMode|UDTSlopeBiasMode|UDTBestPrecisionMode}{g=UDTSignedSign|UDTUnsignedSign}),min,max,unidt({a=36|34|35|}{i=Inherit: Inherit via internal rule|Inherit: Same as input}{b=double|single|int8|uint8|int16|uint16|int32|uint32}{s=UDTBinaryPointMode|UDTSlopeBiasMode|UDTBestPrecisionMode}{g=UDTSignedSign|UDTUnsignedSign}),min,max,unidt({a=39|37|38|}{i=Inherit: Inherit via internal rule|Inherit: Same as input}{b=double|single|int8|uint8|int16|uint16|int32|uint32}{s=UDTBinaryPointMode|UDTSlopeBiasMode|UDTBestPrecisionMode}{g=UDTSignedSign|UDTUnsignedSign}),min,max,unidt({a=42|40|41|}{i=Inherit: Inherit via internal rule|Inherit: Same as input}{b=double|single|int8|uint8|int16|uint16|int32|uint32}{s=UDTBinaryPointMode|UDTSlopeBiasMode|UDTBestPrecisionMode}{g=UDTSignedSign|UDTUnsignedSign}),min,max,unidt({a=45|43|44|}{i=Inherit: Inherit via internal rule|Inherit: Same as input}{b=double|single|int8|uint8|int16|uint16|int32|uint32}{s=UDTBinaryPointMode|UDTSlopeBiasMode|UDTBestPrecisionMode}{g=UDTSignedSign|UDTUnsignedSign}),min,max,unidt({a=48|46|47|}{i=Inherit: Inherit via internal rule|Inherit: Inherit via back propagation|Inherit: Same as input}{b=double|single|int8|uint8|int16|uint16|int32|uint32}{s=UDTBinaryPointMode|UDTSlopeBiasMode}{g=UDTSignedSign|UDTUnsignedSign}),min,max,unidt({a=51|49|50|}{i=Inherit: Inherit via internal rule|Inherit: Inherit via back propagation|Inherit: Same as input}{b=double|single|int8|uint8|int16|uint16|int32|uint32}{s=UDTBinaryPointMode|UDTSlopeBiasMode}{g=UDTSignedSign|UDTUnsignedSign}),min,max,unidt({a=54|52|53|}{i=Inherit: Inherit via internal rule|Inherit: Inherit via back propagation|Inherit: Same as input}{b=double|single|int8|uint8|int16|uint16|int32|uint32}{s=UDTBinaryPointMode|UDTSlopeBiasMode}{g=UDTSignedSign|UDTUnsignedSign}),min,max,unidt({a=57|55|56|}{i=Inherit: Inherit via internal rule|Inherit: Inherit via back propagation|Inherit: Same as input}{b=double|single|int8|uint8|int16|uint16|int32|uint32}{s=UDTBinaryPointMode|UDTSlopeBiasMode}{g=UDTSignedSign|UDTUnsignedSign}),min,max,unidt({a=60|58|59|}{i=Inherit: Inherit via internal rule|Inherit: Inherit via back propagation|Inherit: Same as input}{b=double|single|int8|uint8|int16|uint16|int32|uint32}{s=UDTBinaryPointMode|UDTSlopeBiasMode}{g=UDTSignedSign|UDTUnsignedSign}),min,max,unidt({a=63|61|62|}{i=Inherit: Inherit via internal rule|Inherit: Inherit via back propagation|Inherit: Same as input}{b=double|single|int8|uint8|int16|uint16|int32|uint32}{s=UDTBinaryPointMode|UDTSlopeBiasMode}{g=UDTSignedSign|UDTUnsignedSign}),min,max,unidt({a=66|64|65|}{i=Inherit: Inherit via internal rule|Inherit: Inherit via back propagation}{b=double|single|int8|uint8|int16|uint16|int32|uint32}{s=UDTBinaryPointMode|UDTSlopeBiasMode}{g=UDTSignedSign|UDTUnsignedSign}),min,max,unidt({a=69|67|68|}{i=Inherit: Inherit via internal rule|Inherit: Inherit via back propagation}{b=double|single|int8|uint8|int16|uint16|int32|uint32}{s=UDTBinaryPointMode|UDTSlopeBiasMode}{g=UDTSignedSign|UDTUnsignedSign}),min,max,unidt({a=72|70|71|}{i=Inherit: Inherit via internal rule|Inherit: Inherit via back propagation|Inherit: Same as first input|Inherit: Same as accumulator}{b=double|single|int8|uint8|int16|uint16|int32|uint32}{s=UDTBinaryPointMode|UDTSlopeBiasMode}{g=UDTSignedSign|UDTUnsignedSign}),min,max,unidt({a=75|73|74|}{i=Inherit: Inherit via internal rule|Inherit: Inherit via back propagation|Inherit: Same as first input|Inherit: Same as accumulator}{b=double|single|int8|uint8|int16|uint16|int32|uint32}{s=UDTBinaryPointMode|UDTSlopeBiasMode}{g=UDTSignedSign|UDTUnsignedSign}),min,max,unidt({a=78|76|77|}{i=Inherit: Inherit via internal rule|Inherit: Inherit via back propagation|Inherit: Same as first input|Inherit: Same as accumulator}{b=double|single|int8|uint8|int16|uint16|int32|uint32}{s=UDTBinaryPointMode|UDTSlopeBiasMode}{g=UDTSignedSign|UDTUnsignedSign}),min,max,unidt({a=81|79|80|}{i=Inherit: Inherit via internal rule|Inherit: Inherit via back propagation|Inherit: Same as first input|Inherit: Same as accumulator}{b=double|single|int8|uint8|int16|uint16|int32|uint32}{s=UDTBinaryPointMode|UDTSlopeBiasMode}{g=UDTSignedSign|UDTUnsignedSign}),min,max,unidt({a=84|82|83|}{i=Inherit: Inherit via internal rule|Inherit: Inherit via back propagation|Inherit: Same as first input|Inherit: Same as accumulator}{b=double|single|int8|uint8|int16|uint16|int32|uint32}{s=UDTBinaryPointMode|UDTSlopeBiasMode}{g=UDTSignedSign|UDTUnsignedSign}),unidt({a=85|||}{i=Inherit: Inherit via internal rule|Inherit: Same as first input}{b=double|single|int8|uint8|int16|uint16|int32|uint32}{s=UDTBinaryPointMode|UDTSlopeBiasMode}{g=UDTSignedSign|UDTUnsignedSign}),unidt({a=86|||}{i=Inherit: Inherit via internal rule|Inherit: Same as first input}{b=double|single|int8|uint8|int16|uint16|int32|uint32}{s=UDTBinaryPointMode|UDTSlopeBiasMode}{g=UDTSignedSign|UDTUnsignedSign}),unidt({a=87|||}{i=Inherit: Inherit via internal rule|Inherit: Same as first input}{b=double|single|int8|uint8|int16|uint16|int32|uint32}{s=UDTBinaryPointMode|UDTSlopeBiasMode}{g=UDTSignedSign|UDTUnsignedSign}),unidt({a=88|||}{i=Inherit: Inherit via internal rule|Inherit: Same as first input}{b=double|single|int8|uint8|int16|uint16|int32|uint32}{s=UDTBinaryPointMode|UDTSlopeBiasMode}{g=UDTSignedSign|UDTUnsignedSign}),unidt({a=89|||}{i=Inherit: Inherit via internal rule|Inherit: Same as first input}{b=double|single|int8|uint8|int16|uint16|int32|uint32}{s=UDTBinaryPointMode|UDTSlopeBiasMode}{g=UDTSignedSign|UDTUnsignedSign}),min,max,unidt({a=92|90|91|}{i=Inherit: Inherit via back propagation|Inherit: Same as input}{b=double|single|int8|uint8|int16|uint16|int32|uint32}{s=UDTBinaryPointMode|UDTSlopeBiasMode}{g=UDTSignedSign|UDTUnsignedSign}),edit,edit,checkbox,popup(Auto|ExportedGlobal|ImportedExtern|ImportedExternPointer),edit,edit,edit,checkbox,popup(Auto|ExportedGlobal|ImportedExtern|ImportedExternPointer),edit
      mask Display:
      | disp('PI(z)')
      | port_label('input',1, '');
      | port_label('output',1, '');plot([0 4 4 7]+2,[0 0 8 8]+8);
      | plot([1 4 6]+2,[3 6 3]+8);
      | plot([0 4 6 10]+32,[0 0 8 8]+18);
  Mux : Mux  Inputs=3
  Mux1 : Mux  Inputs=2
  Saturation : Saturate  UpperLimit=30*pi/180  LowerLimit=-30*pi/180
  Saturation1 : Saturate
  Selector1 : Selector  InputPortWidth=3  IndexOptions=Index vector (dialog)  Indices=[1 2]  OutputSizes=1
  Selector2 : Selector  InputPortWidth=3  IndexOptions=Index vector (dialog)  Indices=[1 2]  OutputSizes=1
  Selector3 : Selector  InputPortWidth=2  IndexOptions=Index vector (dialog)  Indices=[1]  OutputSizes=1
  Selector4 : Selector  InputPortWidth=2  IndexOptions=Index vector (dialog)  Indices=[2]  OutputSizes=1
  Selector5 : Selector  InputPortWidth=3  IndexOptions=Index vector (dialog)  Indices=[3]  OutputSizes=1
  Selector7 : Selector  InputPortWidth=8  IndexOptions=Index vector (dialog)  Indices=[5]  OutputSizes=1
  Sum : Sum  Inputs=|-+
  RPY : Outport
  wires:
  Sum/1 -> Horizontal Velocity/1(u)  "North_error East_error"
  Bus Selector/1 -> Selector1/1  "<velocity>"
  Bus Selector/2 -> Selector2/1  "<velocity des>"
  Selector1/1 -> Sum/1
  Selector2/1 -> Sum/2
  UAV Bus/1 -> Bus Selector/1, Bus Selector3/1, Bus Selector1/1
  Horizontal Velocity/1(y) -> Selector3/1, Selector4/1  "North Command East Command"
  Bus Selector1/1 -> Selector5/1  "<attitude>"
  Selector3/1 -> Mux/1
  Selector4/1 -> Mux/2
  Selector5/1 -> Mux/3
  Mux/1 -> Fcn/1, Fcn1/1
  Fcn1/1 -> Saturation/1
  Fcn/1 -> Saturation1/1
  Saturation/1 -> Mux1/1  "desired Roll"
  Saturation1/1 -> Mux1/2  "desired Pitch"
  Mux1/1 -> Gain/1
  Gain/1 -> RPY/1
  Bus Selector3/1 -> Selector7/1  "<rc>"
  Selector7/1 -> Horizontal Velocity/2(RESET)  "reset"

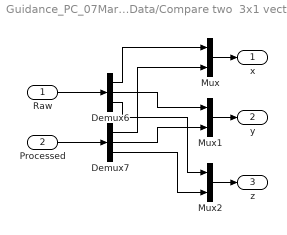
== system Guidance_PC_07Mar2013/Vicon_Data/Compare two  3x1 vectors ==
  Raw : Inport
  Processed : Inport  Port=2
  Demux6 : Demux  Outputs=3
  Demux7 : Demux  Outputs=3
  Mux : Mux  Inputs=2
  Mux1 : Mux  Inputs=2
  Mux2 : Mux  Inputs=2
  x : Outport
  y : Outport  Port=2
  z : Outport  Port=3
  wires:
  Demux6/1 -> Mux/1
  Demux6/2 -> Mux1/1
  Demux7/2 -> Mux1/2
  Demux6/3 -> Mux2/1
  Demux7/3 -> Mux2/2
  Raw/1 -> Demux6/1
  Processed/1 -> Demux7/1
  Mux/1 -> x/1
  Mux1/1 -> y/1
  Mux2/1 -> z/1
  Demux7/1 -> Mux/2

== system Guidance_PC_07Mar2013/Vicon_Data/Compare two  3x1 vectors1 ==
  Raw : Inport
  Processed : Inport  Port=2
  Demux6 : Demux  Outputs=3
  Demux7 : Demux  Outputs=3
  Mux : Mux  Inputs=2
  Mux1 : Mux  Inputs=2
  Mux2 : Mux  Inputs=2
  roll : Outport
  pitch : Outport  Port=2
  yaw : Outport  Port=3
  wires:
  Demux7/1 -> Mux/2
  Mux2/1 -> yaw/1
  Mux1/1 -> pitch/1
  Mux/1 -> roll/1
  Processed/1 -> Demux7/1
  Raw/1 -> Demux6/1
  Demux7/3 -> Mux2/2
  Demux6/3 -> Mux2/1
  Demux7/2 -> Mux1/2
  Demux6/2 -> Mux1/1
  Demux6/1 -> Mux/1

== system Guidance_PC_07Mar2013/Vicon_Data/Low Pass Filter ==
  In1 : Inport
  Gain : Gain  Gain=8
  Integrator : Integrator
  Sum : Sum  Inputs=|+-
  Pos : Outport
  Vel : Outport  Port=2
  wires:
  Sum/1 -> Gain/1
  Gain/1 -> Integrator/1, Vel/1
  Integrator/1 -> Pos/1, Sum/2
  In1/1 -> Sum/1

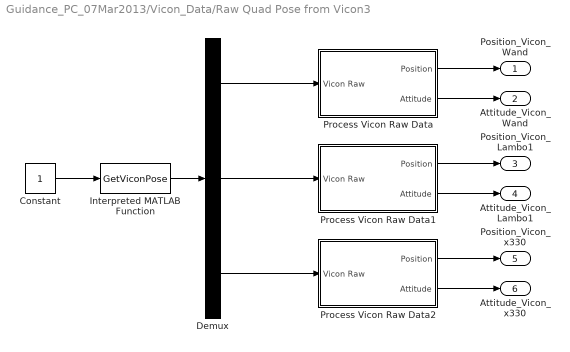
== system Guidance_PC_07Mar2013/Vicon_Data/Raw Quad Pose from Vicon3 ==
  Constant : Constant
  Demux : Demux  Outputs=3
  Interpreted MATLAB Function : MATLABFcn  MATLABFcn=GetViconPose
  Process Vicon Raw Data : Subsystem
  Process Vicon Raw Data1 : Subsystem
  Process Vicon Raw Data2 : Subsystem
  Position_Vicon_Wand : Outport
  Attitude_Vicon_Wand : Outport  Port=2
  Position_Vicon_Lambo1 : Outport  Port=3
  Attitude_Vicon_Lambo1 : Outport  Port=4
  Position_Vicon_x330 : Outport  Port=5
  Attitude_Vicon_x330 : Outport  Port=6
  wires:
  Process Vicon Raw Data/2(Attitude) -> Attitude_Vicon_Wand/1
  Process Vicon Raw Data/1(Position) -> Position_Vicon_Wand/1
  Process Vicon Raw Data1/2(Attitude) -> Attitude_Vicon_Lambo1/1
  Process Vicon Raw Data1/1(Position) -> Position_Vicon_Lambo1/1
  Process Vicon Raw Data2/2(Attitude) -> Attitude_Vicon_x330/1
  Process Vicon Raw Data2/1(Position) -> Position_Vicon_x330/1
  Constant/1 -> Interpreted MATLAB Function/1
  Interpreted MATLAB Function/1 -> Demux/1
  Demux/1 -> Process Vicon Raw Data/1(Vicon Raw)
  Demux/2 -> Process Vicon Raw Data1/1(Vicon Raw)
  Demux/3 -> Process Vicon Raw Data2/1(Vicon Raw)
